simulink model "SimForSecondOrderSystem"  (R2019b)
settings: Solver=VariableStepAuto  StartTime=0.0  StopTime=10  RelTol=1e-6
libraries: dsparch4 x12
settings Model: Creator=19398  LastModifiedBy=19398

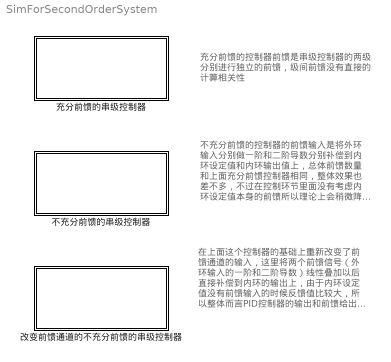
== system SimForSecondOrderSystem ==
  note: 在上面这个控制器的基础上重新改变了前
      | 馈通道的输入，这里将两个前馈信号（外
      | 环输入的一阶和二阶导数）线性叠加以后
      | 直接补偿到内环的输出上，由于内环设定
      | 值没有前馈输入的时候反馈值比较大，所
      | 以整体而言PID控制器的输出和前馈给出
      | 的数据符号相反所以该行为在原理上会降
      | 低控制器性能
  note: 不充分前馈的控制器的前馈输入是将外环
      | 输入分别做一阶和二阶导数分别补偿到内
      | 环设定值和内环输出值上，总体前馈数量
      | 和上面充分前馈控制器相同，整体效果也
      | 差不多，不过在控制环节里面没有考虑内
      | 环设定值本身的前馈所以理论上会稍微降
      | 低控制器性能
  note: 充分前馈的控制器前馈是串级控制器的两级
      | 分别进行独立的前馈，级间前馈没有直接的
      | 计算相关性
  不充分前馈的串级控制器 : Subsystem
  充分前馈的串级控制器 : Subsystem
  改变前馈通道的不充分前馈的串级控制器 : Subsystem

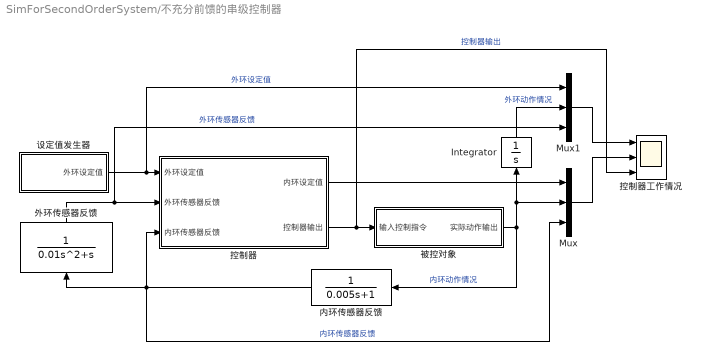
== system SimForSecondOrderSystem/不充分前馈的串级控制器 ==
  Integrator : Integrator
  Mux : Mux  Inputs=3
  Mux1 : Mux  Inputs=3
  内环传感器反馈 : TransferFcn  Denominator=[0.005 1]
  外环传感器反馈 : TransferFcn  Denominator=[0.01 1 0]
  控制器 : Subsystem
  控制器工作情况 : Scope  NumInputPorts=3
  被控对象 : Subsystem
  设定值发生器 : Subsystem
  wires:
  外环传感器反馈/1 -> Mux1/3, 控制器/2(外环传感器反馈)  "外环传感器反馈"
  被控对象/1(实际动作输出) -> 内环传感器反馈/1, Mux/2, Integrator/1  "内环动作情况"
  控制器/2(控制器输出) -> 控制器工作情况/3, 被控对象/1(输入控制指令)  "控制器输出"
  内环传感器反馈/1 -> Mux/3, 外环传感器反馈/1, 控制器/3(内环传感器反馈)  "内环传感器反馈"
  控制器/1(内环设定值) -> Mux/1
  设定值发生器/1(外环设定值) -> Mux1/1, 控制器/1(外环设定值)  "外环设定值"
  Integrator/1 -> Mux1/2  "外环动作情况"
  Mux/1 -> 控制器工作情况/2
  Mux1/1 -> 控制器工作情况/1

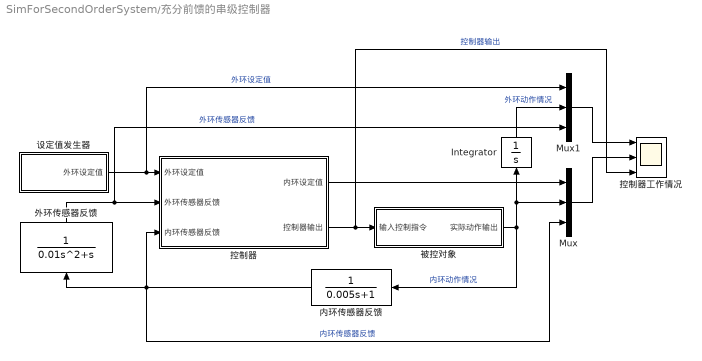
== system SimForSecondOrderSystem/充分前馈的串级控制器 ==
  Integrator : Integrator
  Mux : Mux  Inputs=3
  Mux1 : Mux  Inputs=3
  内环传感器反馈 : TransferFcn  Denominator=[0.005 1]
  外环传感器反馈 : TransferFcn  Denominator=[0.01 1 0]
  控制器 : Subsystem
  控制器工作情况 : Scope  NumInputPorts=3
  被控对象 : Subsystem
  设定值发生器 : Subsystem
  wires:
  外环传感器反馈/1 -> Mux1/3, 控制器/2(外环传感器反馈)  "外环传感器反馈"
  被控对象/1(实际动作输出) -> 内环传感器反馈/1, Mux/2, Integrator/1  "内环动作情况"
  控制器/2(控制器输出) -> 控制器工作情况/3, 被控对象/1(输入控制指令)  "控制器输出"
  内环传感器反馈/1 -> Mux/3, 外环传感器反馈/1, 控制器/3(内环传感器反馈)  "内环传感器反馈"
  控制器/1(内环设定值) -> Mux/1
  设定值发生器/1(外环设定值) -> Mux1/1, 控制器/1(外环设定值)  "外环设定值"
  Integrator/1 -> Mux1/2  "外环动作情况"
  Mux/1 -> 控制器工作情况/2
  Mux1/1 -> 控制器工作情况/1

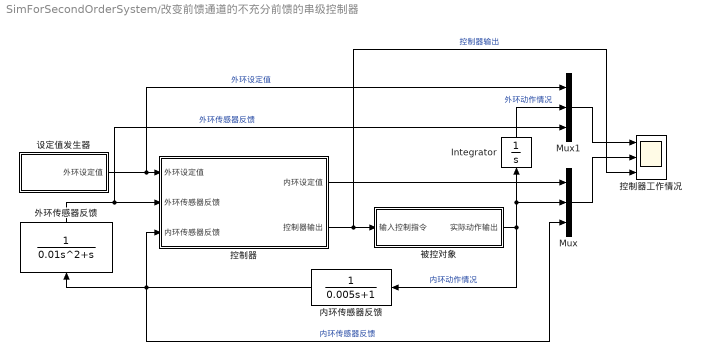
== system SimForSecondOrderSystem/改变前馈通道的不充分前馈的串级控制器 ==
  Integrator : Integrator
  Mux : Mux  Inputs=3
  Mux1 : Mux  Inputs=3
  内环传感器反馈 : TransferFcn  Denominator=[0.005 1]
  外环传感器反馈 : TransferFcn  Denominator=[0.01 1 0]
  控制器 : Subsystem
  控制器工作情况 : Scope  NumInputPorts=3
  被控对象 : Subsystem
  设定值发生器 : Subsystem
  wires:
  外环传感器反馈/1 -> Mux1/3, 控制器/2(外环传感器反馈)  "外环传感器反馈"
  被控对象/1(实际动作输出) -> 内环传感器反馈/1, Mux/2, Integrator/1  "内环动作情况"
  控制器/2(控制器输出) -> 控制器工作情况/3, 被控对象/1(输入控制指令)  "控制器输出"
  内环传感器反馈/1 -> Mux/3, 外环传感器反馈/1, 控制器/3(内环传感器反馈)  "内环传感器反馈"
  控制器/1(内环设定值) -> Mux/1
  设定值发生器/1(外环设定值) -> Mux1/1, 控制器/1(外环设定值)  "外环设定值"
  Integrator/1 -> Mux1/2  "外环动作情况"
  Mux/1 -> 控制器工作情况/2
  Mux1/1 -> 控制器工作情况/1

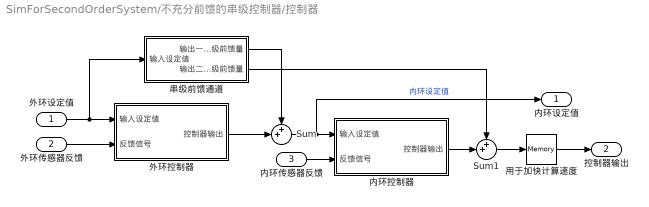
== system SimForSecondOrderSystem/不充分前馈的串级控制器/控制器 ==
  外环设定值 : Inport
  外环传感器反馈 : Inport  Port=2
  内环传感器反馈 : Inport  Port=3
  Sum : Sum  Inputs=++|
  Sum1 : Sum  Inputs=++|
  串级前馈通道 : Subsystem  mask{FrontFeedFilterFreq1=500, FrontFeedFilterFreq2=500, FrontFeedFilterOrder1=8, FrontFeedFilterOrder2=8, K1=1, K2=1, c1=300, c2=300}
      mask prompts: FrontFeedFilterFreq1 "一级前馈输入滤波器截止频率Hz"; FrontFeedFilterFreq2 "二级前馈输入滤波器截止频率Hz"; FrontFeedFilterOrder1 "一级前馈输入滤波器阶数"; FrontFeedFilterOrder2 "二级前馈输入滤波器阶数"; K1 "一级前馈信号增益"; K2 "二级前馈信号增益"; c1 "一级前馈实际微分系数"; c2 "二级前馈实际微分系数"
  内环控制器 : Subsystem
  外环控制器 : Subsystem
  用于加快计算速度 : Memory
  内环设定值 : Outport
  控制器输出 : Outport  Port=2
  wires:
  内环传感器反馈/1 -> 内环控制器/2(反馈信号)
  外环设定值/1 -> 串级前馈通道/1(输入设定值), 外环控制器/1(输入设定值)
  用于加快计算速度/1 -> 控制器输出/1
  外环传感器反馈/1 -> 外环控制器/2(反馈信号)
  外环控制器/1(控制器输出) -> Sum/2
  Sum/1 -> 内环设定值/1, 内环控制器/1(输入设定值)  "内环设定值"
  内环控制器/1(控制器输出) -> Sum1/2
  Sum1/1 -> 用于加快计算速度/1
  串级前馈通道/1(输出一级前馈量) -> Sum/1
  串级前馈通道/2(输出二级前馈量) -> Sum1/1

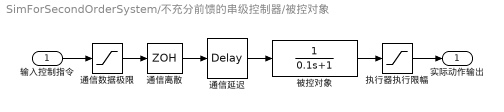
== system SimForSecondOrderSystem/不充分前馈的串级控制器/被控对象 ==
  输入控制指令 : Inport
  执行器执行限幅 : Saturate  UpperLimit=20  LowerLimit=-20
  被控对象 : TransferFcn  Denominator=[0.1 1]
  通信延迟 : TransportDelay  DelayTime=0.001
  通信数据极限 : Saturate  UpperLimit=20  LowerLimit=-20
  通信离散 : ZeroOrderHold  SampleTime=0.001
  实际动作输出 : Outport
  wires:
  被控对象/1 -> 执行器执行限幅/1
  输入控制指令/1 -> 通信数据极限/1
  通信延迟/1 -> 被控对象/1
  通信离散/1 -> 通信延迟/1
  通信数据极限/1 -> 通信离散/1
  执行器执行限幅/1 -> 实际动作输出/1

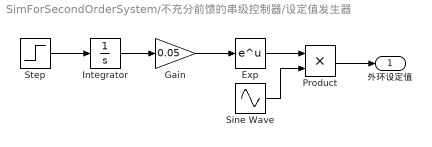
== system SimForSecondOrderSystem/不充分前馈的串级控制器/设定值发生器 ==
  Exp : Math  SignedPower=off  SaturateOnIntegerOverflow=on
  Gain : Gain  Gain=0.05
  Integrator : Integrator
  Product : Product
  Sine Wave : Sin  Frequency=5  SampleTime=0
  Step : Step  Time=0  SampleTime=0
  外环设定值 : Outport
  wires:
  Product/1 -> 外环设定值/1
  Gain/1 -> Exp/1
  Integrator/1 -> Gain/1
  Sine Wave/1 -> Product/2
  Step/1 -> Integrator/1
  Exp/1 -> Product/1

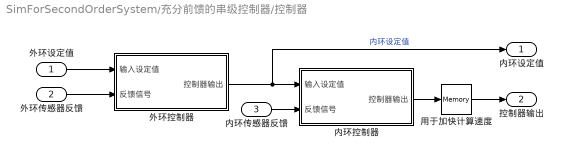
== system SimForSecondOrderSystem/充分前馈的串级控制器/控制器 ==
  外环设定值 : Inport
  外环传感器反馈 : Inport  Port=2
  内环传感器反馈 : Inport  Port=3
  内环控制器 : Subsystem
  外环控制器 : Subsystem
  用于加快计算速度 : Memory
  内环设定值 : Outport
  控制器输出 : Outport  Port=2
  wires:
  内环传感器反馈/1 -> 内环控制器/2(反馈信号)
  外环控制器/1(控制器输出) -> 内环设定值/1, 内环控制器/1(输入设定值)  "内环设定值"
  外环设定值/1 -> 外环控制器/1(输入设定值)
  内环控制器/1(控制器输出) -> 用于加快计算速度/1
  用于加快计算速度/1 -> 控制器输出/1
  外环传感器反馈/1 -> 外环控制器/2(反馈信号)

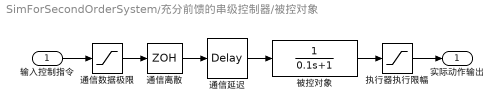
== system SimForSecondOrderSystem/充分前馈的串级控制器/被控对象 ==
  输入控制指令 : Inport
  执行器执行限幅 : Saturate  UpperLimit=20  LowerLimit=-20
  被控对象 : TransferFcn  Denominator=[0.1 1]
  通信延迟 : TransportDelay  DelayTime=0.001
  通信数据极限 : Saturate  UpperLimit=20  LowerLimit=-20
  通信离散 : ZeroOrderHold  SampleTime=0.001
  实际动作输出 : Outport
  wires:
  被控对象/1 -> 执行器执行限幅/1
  输入控制指令/1 -> 通信数据极限/1
  通信延迟/1 -> 被控对象/1
  通信离散/1 -> 通信延迟/1
  通信数据极限/1 -> 通信离散/1
  执行器执行限幅/1 -> 实际动作输出/1

== system SimForSecondOrderSystem/充分前馈的串级控制器/设定值发生器 ==
  Exp : Math  SignedPower=off  SaturateOnIntegerOverflow=on
  Gain : Gain  Gain=0.05
  Integrator : Integrator
  Product : Product
  Sine Wave : Sin  Frequency=5  SampleTime=0
  Step : Step  Time=0  SampleTime=0
  外环设定值 : Outport
  wires:
  Product/1 -> 外环设定值/1
  Gain/1 -> Exp/1
  Integrator/1 -> Gain/1
  Sine Wave/1 -> Product/2
  Step/1 -> Integrator/1
  Exp/1 -> Product/1

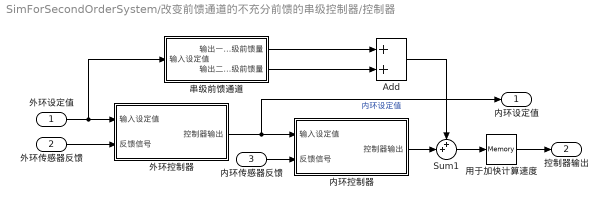
== system SimForSecondOrderSystem/改变前馈通道的不充分前馈的串级控制器/控制器 ==
  外环设定值 : Inport
  外环传感器反馈 : Inport  Port=2
  内环传感器反馈 : Inport  Port=3
  Add : Sum
  Sum1 : Sum  Inputs=++|
  串级前馈通道 : Subsystem  mask{FrontFeedFilterFreq1=500, FrontFeedFilterFreq2=500, FrontFeedFilterOrder1=8, FrontFeedFilterOrder2=8, K1=1.2, K2=1, c1=300, c2=300}
      mask prompts: FrontFeedFilterFreq1 "一级前馈输入滤波器截止频率Hz"; FrontFeedFilterFreq2 "二级前馈输入滤波器截止频率Hz"; FrontFeedFilterOrder1 "一级前馈输入滤波器阶数"; FrontFeedFilterOrder2 "二级前馈输入滤波器阶数"; K1 "一级前馈信号增益"; K2 "二级前馈信号增益"; c1 "一级前馈实际微分系数"; c2 "二级前馈实际微分系数"
  内环控制器 : Subsystem
  外环控制器 : Subsystem
  用于加快计算速度 : Memory
  内环设定值 : Outport
  控制器输出 : Outport  Port=2
  wires:
  内环传感器反馈/1 -> 内环控制器/2(反馈信号)
  外环设定值/1 -> 串级前馈通道/1(输入设定值), 外环控制器/1(输入设定值)
  用于加快计算速度/1 -> 控制器输出/1
  外环传感器反馈/1 -> 外环控制器/2(反馈信号)
  外环控制器/1(控制器输出) -> 内环控制器/1(输入设定值), 内环设定值/1  "内环设定值"
  内环控制器/1(控制器输出) -> Sum1/2
  Sum1/1 -> 用于加快计算速度/1
  串级前馈通道/2(输出二级前馈量) -> Add/2
  Add/1 -> Sum1/1
  串级前馈通道/1(输出一级前馈量) -> Add/1

== system SimForSecondOrderSystem/改变前馈通道的不充分前馈的串级控制器/被控对象 ==
  输入控制指令 : Inport
  执行器执行限幅 : Saturate  UpperLimit=20  LowerLimit=-20
  被控对象 : TransferFcn  Denominator=[0.1 1]
  通信延迟 : TransportDelay  DelayTime=0.001
  通信数据极限 : Saturate  UpperLimit=20  LowerLimit=-20
  通信离散 : ZeroOrderHold  SampleTime=0.001
  实际动作输出 : Outport
  wires:
  被控对象/1 -> 执行器执行限幅/1
  输入控制指令/1 -> 通信数据极限/1
  通信延迟/1 -> 被控对象/1
  通信离散/1 -> 通信延迟/1
  通信数据极限/1 -> 通信离散/1
  执行器执行限幅/1 -> 实际动作输出/1

== system SimForSecondOrderSystem/改变前馈通道的不充分前馈的串级控制器/设定值发生器 ==
  Exp : Math  SignedPower=off  SaturateOnIntegerOverflow=on
  Gain : Gain  Gain=0.05
  Integrator : Integrator
  Product : Product
  Sine Wave : Sin  Frequency=5  SampleTime=0
  Step : Step  Time=0  SampleTime=0
  外环设定值 : Outport
  wires:
  Product/1 -> 外环设定值/1
  Gain/1 -> Exp/1
  Integrator/1 -> Gain/1
  Sine Wave/1 -> Product/2
  Step/1 -> Integrator/1
  Exp/1 -> Product/1

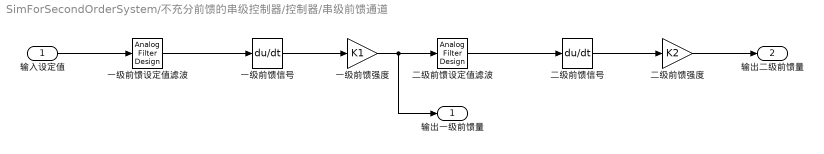
== system SimForSecondOrderSystem/不充分前馈的串级控制器/控制器/串级前馈通道 ==
  输入设定值 : Inport
  一级前馈信号 : Derivative  CoefficientInTFapproximation=c1
  一级前馈强度 : Gain  Gain=K1
  一级前馈设定值滤波 : dsparch4/Analog Filter Design  method=Butterworth  filttype=Lowpass  N=FrontFeedFilterOrder1  Wlo=FrontFeedFilterFreq1*2*pi  Whi=80  Rp=2  Rs=40
  二级前馈信号 : Derivative  CoefficientInTFapproximation=c2
  二级前馈强度 : Gain  Gain=K2
  二级前馈设定值滤波 : dsparch4/Analog Filter Design  method=Butterworth  filttype=Lowpass  N=FrontFeedFilterOrder2  Wlo=FrontFeedFilterFreq2*2*pi  Whi=80  Rp=2  Rs=40
  输出一级前馈量 : Outport
  输出二级前馈量 : Outport  Port=2
  wires:
  一级前馈信号/1 -> 一级前馈强度/1
  二级前馈强度/1 -> 输出二级前馈量/1
  一级前馈设定值滤波/1 -> 一级前馈信号/1
  二级前馈设定值滤波/1 -> 二级前馈信号/1
  二级前馈信号/1 -> 二级前馈强度/1
  输入设定值/1 -> 一级前馈设定值滤波/1
  一级前馈强度/1 -> 输出一级前馈量/1, 二级前馈设定值滤波/1

== system SimForSecondOrderSystem/不充分前馈的串级控制器/控制器/内环控制器 ==
  输入设定值 : Inport
  反馈信号 : Inport  Port=2
  Sum : Sum  Inputs=|+-
  内环PID控制器 : Subsystem  mask{Kp=50, Ki=5, iLimit=1, Kd=0.035, c=500, DFilterOrder=6, DFilterFreq=300, OutLim=50}
      mask prompts: Kp "比例增益系数"; Ki "积分增益系数"; iLimit "积分限幅"; Kd "微分增益系数"; c "实际微分系数"; DFilterOrder "微分滤波器阶数"; DFilterFreq "微分滤波器截止频率Hz"; OutLim "输出限幅"
  控制器输出 : Outport
  wires:
  内环PID控制器/1(控制器输出) -> 控制器输出/1
  Sum/1 -> 内环PID控制器/1(输入误差)
  输入设定值/1 -> Sum/1
  反馈信号/1 -> Sum/2

== system SimForSecondOrderSystem/不充分前馈的串级控制器/控制器/外环控制器 ==
  输入设定值 : Inport
  反馈信号 : Inport  Port=2
  Sum : Sum  Inputs=|+-
  外环PID控制器 : Subsystem  mask{Kp=1, Ki=0.01, iLimit=5, Kd=0, c=500, DFilterOrder=6, DFilterFreq=300, OutLim=50}
      mask prompts: Kp "比例增益系数"; Ki "积分增益系数"; iLimit "积分限幅"; Kd "微分增益系数"; c "实际微分系数"; DFilterOrder "微分滤波器阶数"; DFilterFreq "微分滤波器截止频率Hz"; OutLim "输出限幅"
  控制器输出 : Outport
  wires:
  外环PID控制器/1(控制器输出) -> 控制器输出/1
  Sum/1 -> 外环PID控制器/1(输入误差)
  输入设定值/1 -> Sum/1
  反馈信号/1 -> Sum/2

== system SimForSecondOrderSystem/充分前馈的串级控制器/控制器/内环控制器 ==
  输入设定值 : Inport
  反馈信号 : Inport  Port=2
  Sum : Sum  Inputs=|+-
  Sum1 : Sum  Inputs=++|
  内环PID控制器 : Subsystem  mask{Kp=50, Ki=5, iLimit=1, Kd=0.035, c=500, DFilterOrder=6, DFilterFreq=300, OutLim=50}
      mask prompts: Kp "比例增益系数"; Ki "积分增益系数"; iLimit "积分限幅"; Kd "微分增益系数"; c "实际微分系数"; DFilterOrder "微分滤波器阶数"; DFilterFreq "微分滤波器截止频率Hz"; OutLim "输出限幅"
  前馈通道 : Subsystem  mask{FrontFeedFilterFreq=500, FrontFeedFilterOrder=8, K=1, c=300}
      mask prompts: FrontFeedFilterFreq "前馈输入滤波器截止频率Hz"; FrontFeedFilterOrder "前馈输入滤波器阶数"; K "前馈信号增益"; c "前馈实际微分系数"
  控制器输出 : Outport
  wires:
  Sum1/1 -> 控制器输出/1
  Sum/1 -> 内环PID控制器/1(输入误差)
  前馈通道/1(输出前馈量) -> Sum1/1
  输入设定值/1 -> Sum/1, 前馈通道/1(输入设定值)
  反馈信号/1 -> Sum/2
  内环PID控制器/1(控制器输出) -> Sum1/2

== system SimForSecondOrderSystem/充分前馈的串级控制器/控制器/外环控制器 ==
  输入设定值 : Inport
  反馈信号 : Inport  Port=2
  Sum : Sum  Inputs=|+-
  Sum1 : Sum  Inputs=++|
  前馈通道 : Subsystem  mask{FrontFeedFilterFreq=500, FrontFeedFilterOrder=8, K=1, c=300}
      mask prompts: FrontFeedFilterFreq "前馈输入滤波器截止频率Hz"; FrontFeedFilterOrder "前馈输入滤波器阶数"; K "前馈信号增益"; c "前馈实际微分系数"
  外环PID控制器 : Subsystem  mask{Kp=1, Ki=0.01, iLimit=5, Kd=0, c=500, DFilterOrder=6, DFilterFreq=300, OutLim=50}
      mask prompts: Kp "比例增益系数"; Ki "积分增益系数"; iLimit "积分限幅"; Kd "微分增益系数"; c "实际微分系数"; DFilterOrder "微分滤波器阶数"; DFilterFreq "微分滤波器截止频率Hz"; OutLim "输出限幅"
  控制器输出 : Outport
  wires:
  Sum1/1 -> 控制器输出/1
  Sum/1 -> 外环PID控制器/1(输入误差)
  前馈通道/1(输出前馈量) -> Sum1/1
  输入设定值/1 -> Sum/1, 前馈通道/1(输入设定值)
  反馈信号/1 -> Sum/2
  外环PID控制器/1(控制器输出) -> Sum1/2

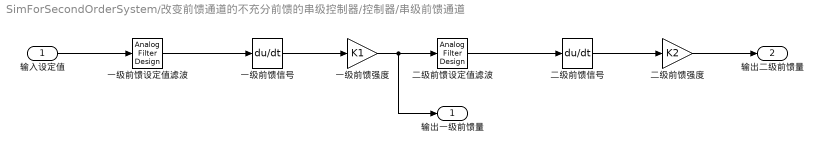
== system SimForSecondOrderSystem/改变前馈通道的不充分前馈的串级控制器/控制器/串级前馈通道 ==
  输入设定值 : Inport
  一级前馈信号 : Derivative  CoefficientInTFapproximation=c1
  一级前馈强度 : Gain  Gain=K1
  一级前馈设定值滤波 : dsparch4/Analog Filter Design  method=Butterworth  filttype=Lowpass  N=FrontFeedFilterOrder1  Wlo=FrontFeedFilterFreq1*2*pi  Whi=80  Rp=2  Rs=40
  二级前馈信号 : Derivative  CoefficientInTFapproximation=c2
  二级前馈强度 : Gain  Gain=K2
  二级前馈设定值滤波 : dsparch4/Analog Filter Design  method=Butterworth  filttype=Lowpass  N=FrontFeedFilterOrder2  Wlo=FrontFeedFilterFreq2*2*pi  Whi=80  Rp=2  Rs=40
  输出一级前馈量 : Outport
  输出二级前馈量 : Outport  Port=2
  wires:
  一级前馈信号/1 -> 一级前馈强度/1
  二级前馈强度/1 -> 输出二级前馈量/1
  一级前馈设定值滤波/1 -> 一级前馈信号/1
  二级前馈设定值滤波/1 -> 二级前馈信号/1
  二级前馈信号/1 -> 二级前馈强度/1
  输入设定值/1 -> 一级前馈设定值滤波/1
  一级前馈强度/1 -> 输出一级前馈量/1, 二级前馈设定值滤波/1

== system SimForSecondOrderSystem/改变前馈通道的不充分前馈的串级控制器/控制器/内环控制器 ==
  输入设定值 : Inport
  反馈信号 : Inport  Port=2
  Sum : Sum  Inputs=|+-
  内环PID控制器 : Subsystem  mask{Kp=50, Ki=5, iLimit=1, Kd=0.035, c=500, DFilterOrder=6, DFilterFreq=300, OutLim=50}
      mask prompts: Kp "比例增益系数"; Ki "积分增益系数"; iLimit "积分限幅"; Kd "微分增益系数"; c "实际微分系数"; DFilterOrder "微分滤波器阶数"; DFilterFreq "微分滤波器截止频率Hz"; OutLim "输出限幅"
  控制器输出 : Outport
  wires:
  内环PID控制器/1(控制器输出) -> 控制器输出/1
  Sum/1 -> 内环PID控制器/1(输入误差)
  输入设定值/1 -> Sum/1
  反馈信号/1 -> Sum/2

== system SimForSecondOrderSystem/改变前馈通道的不充分前馈的串级控制器/控制器/外环控制器 ==
  输入设定值 : Inport
  反馈信号 : Inport  Port=2
  Sum : Sum  Inputs=|+-
  外环PID控制器 : Subsystem  mask{Kp=1, Ki=0.01, iLimit=5, Kd=0, c=500, DFilterOrder=6, DFilterFreq=300, OutLim=50}
      mask prompts: Kp "比例增益系数"; Ki "积分增益系数"; iLimit "积分限幅"; Kd "微分增益系数"; c "实际微分系数"; DFilterOrder "微分滤波器阶数"; DFilterFreq "微分滤波器截止频率Hz"; OutLim "输出限幅"
  控制器输出 : Outport
  wires:
  外环PID控制器/1(控制器输出) -> 控制器输出/1
  Sum/1 -> 外环PID控制器/1(输入误差)
  输入设定值/1 -> Sum/1
  反馈信号/1 -> Sum/2

== system SimForSecondOrderSystem/不充分前馈的串级控制器/控制器/内环控制器/内环PID控制器 ==
  输入误差 : Inport
  Sum : Sum  Inputs=+++
  微分环节 : Subsystem  mask{Kd=Kd, c=c, DFilterOrder=DFilterOrder, DFilterFreq=DFilterFreq}
      mask prompts: Kd "微分增益系数"; c "实际微分系数"; DFilterOrder "微分滤波器阶数"; DFilterFreq "微分滤波器截止频率Hz"
  比例环节 : Subsystem  mask{Kp=Kp}
      mask prompts: Kp "比例增益系数"
  积分环节 : Subsystem  mask{Ki=Ki, iLimit=iLimit}
      mask prompts: Ki "积分增益系数"; iLimit "积分限幅"
  输出限幅 : Saturate  UpperLimit=OutLim  LowerLimit=-OutLim
  控制器输出 : Outport
  wires:
  输入误差/1 -> 积分环节/1(误差), 微分环节/1(误差), 比例环节/1(误差)
  积分环节/1(积分环节输出) -> Sum/2
  比例环节/1(比例环节输出) -> Sum/1
  微分环节/1(微分环节输出) -> Sum/3
  Sum/1 -> 输出限幅/1
  输出限幅/1 -> 控制器输出/1

== system SimForSecondOrderSystem/不充分前馈的串级控制器/控制器/外环控制器/外环PID控制器 ==
  输入误差 : Inport
  Sum : Sum  Inputs=+++
  微分环节 : Subsystem  mask{Kd=Kd, c=c, DFilterOrder=DFilterOrder, DFilterFreq=DFilterFreq}
      mask prompts: Kd "微分增益系数"; c "实际微分系数"; DFilterOrder "微分滤波器阶数"; DFilterFreq "微分滤波器截止频率Hz"
  比例环节 : Subsystem  mask{Kp=Kp}
      mask prompts: Kp "比例增益系数"
  积分环节 : Subsystem  mask{Ki=Ki, iLimit=iLimit}
      mask prompts: Ki "积分增益系数"; iLimit "积分限幅"
  输出限幅 : Saturate  UpperLimit=OutLim  LowerLimit=-OutLim
  控制器输出 : Outport
  wires:
  输入误差/1 -> 积分环节/1(误差), 微分环节/1(误差), 比例环节/1(误差)
  积分环节/1(积分环节输出) -> Sum/2
  比例环节/1(比例环节输出) -> Sum/1
  微分环节/1(微分环节输出) -> Sum/3
  Sum/1 -> 输出限幅/1
  输出限幅/1 -> 控制器输出/1

== system SimForSecondOrderSystem/充分前馈的串级控制器/控制器/内环控制器/内环PID控制器 ==
  输入误差 : Inport
  Sum : Sum  Inputs=+++
  微分环节 : Subsystem  mask{Kd=Kd, c=c, DFilterOrder=DFilterOrder, DFilterFreq=DFilterFreq}
      mask prompts: Kd "微分增益系数"; c "实际微分系数"; DFilterOrder "微分滤波器阶数"; DFilterFreq "微分滤波器截止频率Hz"
  比例环节 : Subsystem  mask{Kp=Kp}
      mask prompts: Kp "比例增益系数"
  积分环节 : Subsystem  mask{Ki=Ki, iLimit=iLimit}
      mask prompts: Ki "积分增益系数"; iLimit "积分限幅"
  输出限幅 : Saturate  UpperLimit=OutLim  LowerLimit=-OutLim
  控制器输出 : Outport
  wires:
  输入误差/1 -> 积分环节/1(误差), 微分环节/1(误差), 比例环节/1(误差)
  积分环节/1(积分环节输出) -> Sum/2
  比例环节/1(比例环节输出) -> Sum/1
  微分环节/1(微分环节输出) -> Sum/3
  Sum/1 -> 输出限幅/1
  输出限幅/1 -> 控制器输出/1

== system SimForSecondOrderSystem/充分前馈的串级控制器/控制器/内环控制器/前馈通道 ==
  输入设定值 : Inport
  前馈信号 : Derivative  CoefficientInTFapproximation=c
  前馈强度 : Gain  Gain=K
  前馈设定值滤波 : dsparch4/Analog Filter Design  method=Butterworth  filttype=Lowpass  N=FrontFeedFilterOrder  Wlo=FrontFeedFilterFreq*2*pi  Whi=80  Rp=2  Rs=40
  输出前馈量 : Outport
  wires:
  输入设定值/1 -> 前馈设定值滤波/1
  前馈设定值滤波/1 -> 前馈信号/1
  前馈信号/1 -> 前馈强度/1
  前馈强度/1 -> 输出前馈量/1

== system SimForSecondOrderSystem/充分前馈的串级控制器/控制器/外环控制器/前馈通道 ==
  输入设定值 : Inport
  前馈信号 : Derivative  CoefficientInTFapproximation=c
  前馈强度 : Gain  Gain=K
  前馈设定值滤波 : dsparch4/Analog Filter Design  method=Butterworth  filttype=Lowpass  N=FrontFeedFilterOrder  Wlo=FrontFeedFilterFreq*2*pi  Whi=80  Rp=2  Rs=40
  输出前馈量 : Outport
  wires:
  输入设定值/1 -> 前馈设定值滤波/1
  前馈设定值滤波/1 -> 前馈信号/1
  前馈信号/1 -> 前馈强度/1
  前馈强度/1 -> 输出前馈量/1

== system SimForSecondOrderSystem/充分前馈的串级控制器/控制器/外环控制器/外环PID控制器 ==
  输入误差 : Inport
  Sum : Sum  Inputs=+++
  微分环节 : Subsystem  mask{Kd=Kd, c=c, DFilterOrder=DFilterOrder, DFilterFreq=DFilterFreq}
      mask prompts: Kd "微分增益系数"; c "实际微分系数"; DFilterOrder "微分滤波器阶数"; DFilterFreq "微分滤波器截止频率Hz"
  比例环节 : Subsystem  mask{Kp=Kp}
      mask prompts: Kp "比例增益系数"
  积分环节 : Subsystem  mask{Ki=Ki, iLimit=iLimit}
      mask prompts: Ki "积分增益系数"; iLimit "积分限幅"
  输出限幅 : Saturate  UpperLimit=OutLim  LowerLimit=-OutLim
  控制器输出 : Outport
  wires:
  输入误差/1 -> 积分环节/1(误差), 微分环节/1(误差), 比例环节/1(误差)
  积分环节/1(积分环节输出) -> Sum/2
  比例环节/1(比例环节输出) -> Sum/1
  微分环节/1(微分环节输出) -> Sum/3
  Sum/1 -> 输出限幅/1
  输出限幅/1 -> 控制器输出/1

== system SimForSecondOrderSystem/改变前馈通道的不充分前馈的串级控制器/控制器/内环控制器/内环PID控制器 ==
  输入误差 : Inport
  Sum : Sum  Inputs=+++
  微分环节 : Subsystem  mask{Kd=Kd, c=c, DFilterOrder=DFilterOrder, DFilterFreq=DFilterFreq}
      mask prompts: Kd "微分增益系数"; c "实际微分系数"; DFilterOrder "微分滤波器阶数"; DFilterFreq "微分滤波器截止频率Hz"
  比例环节 : Subsystem  mask{Kp=Kp}
      mask prompts: Kp "比例增益系数"
  积分环节 : Subsystem  mask{Ki=Ki, iLimit=iLimit}
      mask prompts: Ki "积分增益系数"; iLimit "积分限幅"
  输出限幅 : Saturate  UpperLimit=OutLim  LowerLimit=-OutLim
  控制器输出 : Outport
  wires:
  输入误差/1 -> 积分环节/1(误差), 微分环节/1(误差), 比例环节/1(误差)
  积分环节/1(积分环节输出) -> Sum/2
  比例环节/1(比例环节输出) -> Sum/1
  微分环节/1(微分环节输出) -> Sum/3
  Sum/1 -> 输出限幅/1
  输出限幅/1 -> 控制器输出/1

== system SimForSecondOrderSystem/改变前馈通道的不充分前馈的串级控制器/控制器/外环控制器/外环PID控制器 ==
  输入误差 : Inport
  Sum : Sum  Inputs=+++
  微分环节 : Subsystem  mask{Kd=Kd, c=c, DFilterOrder=DFilterOrder, DFilterFreq=DFilterFreq}
      mask prompts: Kd "微分增益系数"; c "实际微分系数"; DFilterOrder "微分滤波器阶数"; DFilterFreq "微分滤波器截止频率Hz"
  比例环节 : Subsystem  mask{Kp=Kp}
      mask prompts: Kp "比例增益系数"
  积分环节 : Subsystem  mask{Ki=Ki, iLimit=iLimit}
      mask prompts: Ki "积分增益系数"; iLimit "积分限幅"
  输出限幅 : Saturate  UpperLimit=OutLim  LowerLimit=-OutLim
  控制器输出 : Outport
  wires:
  输入误差/1 -> 积分环节/1(误差), 微分环节/1(误差), 比例环节/1(误差)
  积分环节/1(积分环节输出) -> Sum/2
  比例环节/1(比例环节输出) -> Sum/1
  微分环节/1(微分环节输出) -> Sum/3
  Sum/1 -> 输出限幅/1
  输出限幅/1 -> 控制器输出/1

== system SimForSecondOrderSystem/不充分前馈的串级控制器/控制器/内环控制器/内环PID控制器/微分环节 ==
  误差 : Inport
  微分器 : Derivative  CoefficientInTFapproximation=c
  微分增益Kd : Gain  Gain=Kd
  微分滤波器 : dsparch4/Analog Filter Design  method=Butterworth  filttype=Lowpass  N=DFilterOrder  Wlo=2*pi*DFilterFreq  Whi=80  Rp=2  Rs=40
  微分环节输出 : Outport
  wires:
  误差/1 -> 微分增益Kd/1
  微分增益Kd/1 -> 微分滤波器/1
  微分器/1 -> 微分环节输出/1
  微分滤波器/1 -> 微分器/1

== system SimForSecondOrderSystem/不充分前馈的串级控制器/控制器/内环控制器/内环PID控制器/比例环节 ==
  误差 : Inport
  比例增益Kp : Gain  Gain=Kp
  比例环节输出 : Outport
  wires:
  误差/1 -> 比例增益Kp/1
  比例增益Kp/1 -> 比例环节输出/1

== system SimForSecondOrderSystem/不充分前馈的串级控制器/控制器/内环控制器/内环PID控制器/积分环节 ==
  误差 : Inport
  积分器 : Integrator
  积分增益Ki : Gain  Gain=Ki
  积分环节的输出 : Scope
  积分限幅 : Saturate  UpperLimit=iLimit  LowerLimit=-iLimit
  积分环节输出 : Outport
  wires:
  误差/1 -> 积分增益Ki/1
  积分增益Ki/1 -> 积分器/1
  积分器/1 -> 积分限幅/1
  积分限幅/1 -> 积分环节的输出/1, 积分环节输出/1

== system SimForSecondOrderSystem/不充分前馈的串级控制器/控制器/外环控制器/外环PID控制器/微分环节 ==
  误差 : Inport
  微分器 : Derivative  CoefficientInTFapproximation=c
  微分增益Kd : Gain  Gain=Kd
  微分滤波器 : dsparch4/Analog Filter Design  method=Butterworth  filttype=Lowpass  N=DFilterOrder  Wlo=2*pi*DFilterFreq  Whi=80  Rp=2  Rs=40
  微分环节输出 : Outport
  wires:
  误差/1 -> 微分增益Kd/1
  微分增益Kd/1 -> 微分滤波器/1
  微分器/1 -> 微分环节输出/1
  微分滤波器/1 -> 微分器/1

== system SimForSecondOrderSystem/不充分前馈的串级控制器/控制器/外环控制器/外环PID控制器/比例环节 ==
  误差 : Inport
  比例增益Kp : Gain  Gain=Kp
  比例环节输出 : Outport
  wires:
  误差/1 -> 比例增益Kp/1
  比例增益Kp/1 -> 比例环节输出/1

== system SimForSecondOrderSystem/不充分前馈的串级控制器/控制器/外环控制器/外环PID控制器/积分环节 ==
  误差 : Inport
  Scope : Scope
  积分器 : Integrator
  积分增益Ki : Gain  Gain=Ki
  积分限幅 : Saturate  UpperLimit=iLimit  LowerLimit=-iLimit
  积分环节输出 : Outport
  wires:
  误差/1 -> 积分增益Ki/1
  积分增益Ki/1 -> 积分器/1
  积分器/1 -> 积分限幅/1
  积分限幅/1 -> Scope/1, 积分环节输出/1

== system SimForSecondOrderSystem/充分前馈的串级控制器/控制器/内环控制器/内环PID控制器/微分环节 ==
  误差 : Inport
  微分器 : Derivative  CoefficientInTFapproximation=c
  微分增益Kd : Gain  Gain=Kd
  微分滤波器 : dsparch4/Analog Filter Design  method=Butterworth  filttype=Lowpass  N=DFilterOrder  Wlo=2*pi*DFilterFreq  Whi=80  Rp=2  Rs=40
  微分环节输出 : Outport
  wires:
  误差/1 -> 微分增益Kd/1
  微分增益Kd/1 -> 微分滤波器/1
  微分器/1 -> 微分环节输出/1
  微分滤波器/1 -> 微分器/1

== system SimForSecondOrderSystem/充分前馈的串级控制器/控制器/内环控制器/内环PID控制器/比例环节 ==
  误差 : Inport
  比例增益Kp : Gain  Gain=Kp
  比例环节输出 : Outport
  wires:
  误差/1 -> 比例增益Kp/1
  比例增益Kp/1 -> 比例环节输出/1

== system SimForSecondOrderSystem/充分前馈的串级控制器/控制器/内环控制器/内环PID控制器/积分环节 ==
  误差 : Inport
  积分器 : Integrator
  积分增益Ki : Gain  Gain=Ki
  积分环节的输出 : Scope
  积分限幅 : Saturate  UpperLimit=iLimit  LowerLimit=-iLimit
  积分环节输出 : Outport
  wires:
  误差/1 -> 积分增益Ki/1
  积分增益Ki/1 -> 积分器/1
  积分器/1 -> 积分限幅/1
  积分限幅/1 -> 积分环节的输出/1, 积分环节输出/1

== system SimForSecondOrderSystem/充分前馈的串级控制器/控制器/外环控制器/外环PID控制器/微分环节 ==
  误差 : Inport
  微分器 : Derivative  CoefficientInTFapproximation=c
  微分增益Kd : Gain  Gain=Kd
  微分滤波器 : dsparch4/Analog Filter Design  method=Butterworth  filttype=Lowpass  N=DFilterOrder  Wlo=2*pi*DFilterFreq  Whi=80  Rp=2  Rs=40
  微分环节输出 : Outport
  wires:
  误差/1 -> 微分增益Kd/1
  微分增益Kd/1 -> 微分滤波器/1
  微分器/1 -> 微分环节输出/1
  微分滤波器/1 -> 微分器/1

== system SimForSecondOrderSystem/充分前馈的串级控制器/控制器/外环控制器/外环PID控制器/比例环节 ==
  误差 : Inport
  比例增益Kp : Gain  Gain=Kp
  比例环节输出 : Outport
  wires:
  误差/1 -> 比例增益Kp/1
  比例增益Kp/1 -> 比例环节输出/1

== system SimForSecondOrderSystem/充分前馈的串级控制器/控制器/外环控制器/外环PID控制器/积分环节 ==
  误差 : Inport
  Scope : Scope
  积分器 : Integrator
  积分增益Ki : Gain  Gain=Ki
  积分限幅 : Saturate  UpperLimit=iLimit  LowerLimit=-iLimit
  积分环节输出 : Outport
  wires:
  误差/1 -> 积分增益Ki/1
  积分增益Ki/1 -> 积分器/1
  积分器/1 -> 积分限幅/1
  积分限幅/1 -> Scope/1, 积分环节输出/1

== system SimForSecondOrderSystem/改变前馈通道的不充分前馈的串级控制器/控制器/内环控制器/内环PID控制器/微分环节 ==
  误差 : Inport
  微分器 : Derivative  CoefficientInTFapproximation=c
  微分增益Kd : Gain  Gain=Kd
  微分滤波器 : dsparch4/Analog Filter Design  method=Butterworth  filttype=Lowpass  N=DFilterOrder  Wlo=2*pi*DFilterFreq  Whi=80  Rp=2  Rs=40
  微分环节输出 : Outport
  wires:
  误差/1 -> 微分增益Kd/1
  微分增益Kd/1 -> 微分滤波器/1
  微分器/1 -> 微分环节输出/1
  微分滤波器/1 -> 微分器/1

== system SimForSecondOrderSystem/改变前馈通道的不充分前馈的串级控制器/控制器/内环控制器/内环PID控制器/比例环节 ==
  误差 : Inport
  比例增益Kp : Gain  Gain=Kp
  比例环节输出 : Outport
  wires:
  误差/1 -> 比例增益Kp/1
  比例增益Kp/1 -> 比例环节输出/1

== system SimForSecondOrderSystem/改变前馈通道的不充分前馈的串级控制器/控制器/内环控制器/内环PID控制器/积分环节 ==
  误差 : Inport
  积分器 : Integrator
  积分增益Ki : Gain  Gain=Ki
  积分环节的输出 : Scope
  积分限幅 : Saturate  UpperLimit=iLimit  LowerLimit=-iLimit
  积分环节输出 : Outport
  wires:
  误差/1 -> 积分增益Ki/1
  积分增益Ki/1 -> 积分器/1
  积分器/1 -> 积分限幅/1
  积分限幅/1 -> 积分环节的输出/1, 积分环节输出/1

== system SimForSecondOrderSystem/改变前馈通道的不充分前馈的串级控制器/控制器/外环控制器/外环PID控制器/微分环节 ==
  误差 : Inport
  微分器 : Derivative  CoefficientInTFapproximation=c
  微分增益Kd : Gain  Gain=Kd
  微分滤波器 : dsparch4/Analog Filter Design  method=Butterworth  filttype=Lowpass  N=DFilterOrder  Wlo=2*pi*DFilterFreq  Whi=80  Rp=2  Rs=40
  微分环节输出 : Outport
  wires:
  误差/1 -> 微分增益Kd/1
  微分增益Kd/1 -> 微分滤波器/1
  微分器/1 -> 微分环节输出/1
  微分滤波器/1 -> 微分器/1

== system SimForSecondOrderSystem/改变前馈通道的不充分前馈的串级控制器/控制器/外环控制器/外环PID控制器/比例环节 ==
  误差 : Inport
  比例增益Kp : Gain  Gain=Kp
  比例环节输出 : Outport
  wires:
  误差/1 -> 比例增益Kp/1
  比例增益Kp/1 -> 比例环节输出/1

== system SimForSecondOrderSystem/改变前馈通道的不充分前馈的串级控制器/控制器/外环控制器/外环PID控制器/积分环节 ==
  误差 : Inport
  Scope : Scope
  积分器 : Integrator
  积分增益Ki : Gain  Gain=Ki
  积分限幅 : Saturate  UpperLimit=iLimit  LowerLimit=-iLimit
  积分环节输出 : Outport
  wires:
  误差/1 -> 积分增益Ki/1
  积分增益Ki/1 -> 积分器/1
  积分器/1 -> 积分限幅/1
  积分限幅/1 -> Scope/1, 积分环节输出/1
